simulink model "SFTimeSignalDemo"  (R2024a)
settings: Solver=FixedStepAuto  StartTime=0.0  StopTime=10.0  RelTol=1e-3
model workspace (MAT data in the model file):
  configPath = Simulink.Parameter
  configPath.Complexity = 'real'
  configPath.Dimensions = [0 0]
  configPath.DataType = 'auto'
settings Model: Creator=deshazere  LastModifiedBy=deshazere
settings RTWCC: GenerateReport=on  LaunchReport=on

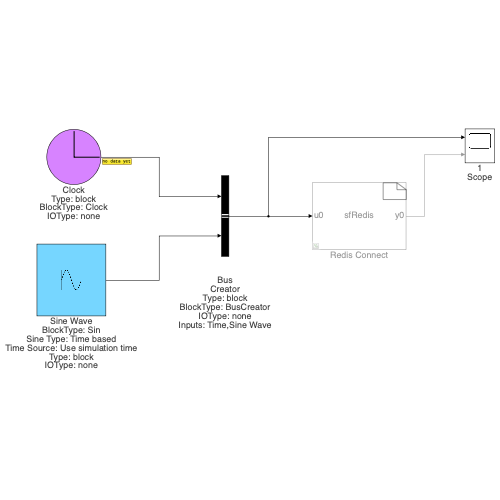
[thumbnail: Simulink's stored preview of the top-level diagram]
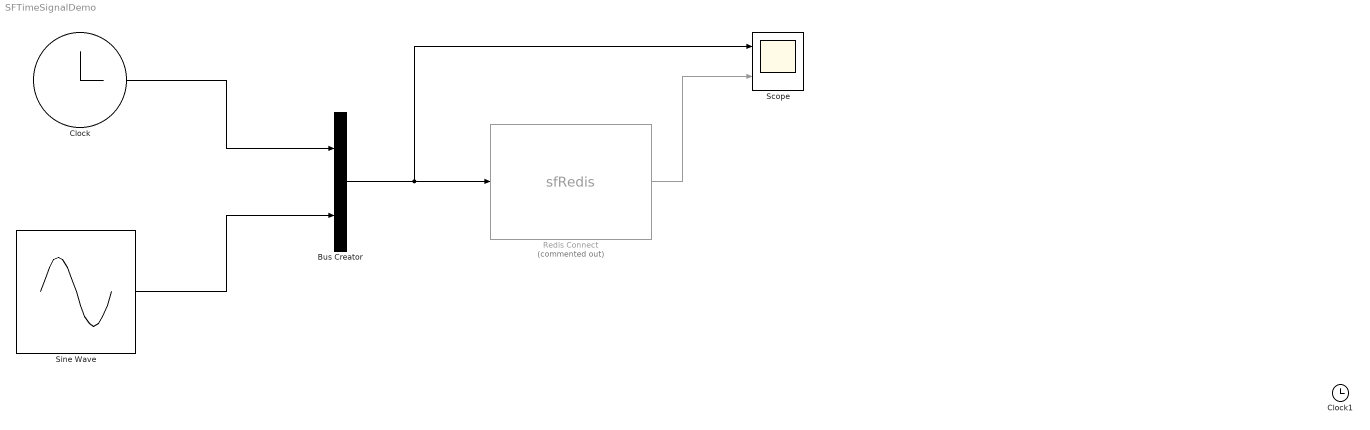
== system SFTimeSignalDemo ==
  Bus Creator : BusCreator  Inputs=Time,Sine Wave  OutDataTypeStr=Bus: sfRedisBus  NonVirtualBus=on
      settings: AttributesFormatString=|
      | %<Name>
      | Type: %<Type>
      | BlockType: %<BlockType>
      | IOType: %<IOType>
      | Inputs: %<Inputs>
  Clock : Clock
      settings: InitFcn=load
      settings: AttributesFormatString=|
      | %<Name>
      | Type: %<Type>
      | BlockType: %<BlockType>
      | IOType: %<IOType>
  Redis Connect : S-Function  Commented=on  FunctionName=sfRedis  Parameters=uint8(1),int32(1),uint8(1)  SFunctionModules=sfRedis_wrapper.c  SFunctionDeploymentMode=off  EnableBusSupport=off  mask(S-Function Builder){}
      mask help: Simulink:masks:SFunctionBuilder_MD
      mask init:
      | val = [[.9  0.75 0.75 1 1 .9 .9 1]',[1 1 0.75 0.75 .9 .9 1 .9]'];try , sys = get_param(gcb,'SfunBuilderFcnName');if isempty(sys), sys = get_param(gcb,'FunctionName'); end,catch, sys = get_param(gcb,'FunctionName'); end
      settings: CopyFcn=set_param(gcbh,'LinkStatus','none')  OpenFcn=sfunctionwizard(gcbh)
      mask Display: plot(val(:,1),val(:,2)),disp(sys),port_label('input',1,'u0'),port_label('output',1,'y0')
  Scope : Scope  NumInputPorts=2
      settings: AttributesFormatString=|
      | %<ActiveDisplayString>
      | %<BlockType>
  Sine Wave : Sin  SampleTime=0
      settings: AttributesFormatString=|
      | %<Name>
      | BlockType: %<BlockType>
      | Sine Type: %<SineType>
      | Time Source: %<TimeSource>
      | Type: %<Type>
      | IOType: %<IOType>
  Clock1 : Clock
      settings: IOType=siggen
  wires:
  Redis Connect/1 -> Scope/2
  Bus Creator/1 -> Redis Connect/1, Scope/1
  Sine Wave/1 -> Bus Creator/2
  Clock/1 -> Bus Creator/1
